simulink model "Exercicio_2_simulink_Vinicius"  (R2015a)
settings: Solver=ode45  StartTime=0.0  StopTime=40  RelTol=1e-3
values from neighbouring files (symbols this model uses):
  B = [zeros(1,d) 0.4 0.6]    [Exercicio_2_Vinicius_Alexandre.m]
  Ts = 1    [Exercicio_2_Vinicius_Alexandre.m]
undefined symbols (not defined in the file or in its folder): At, D, ke, kf, kw
settings Model: Creator=vinic  LastModifiedBy=vinic

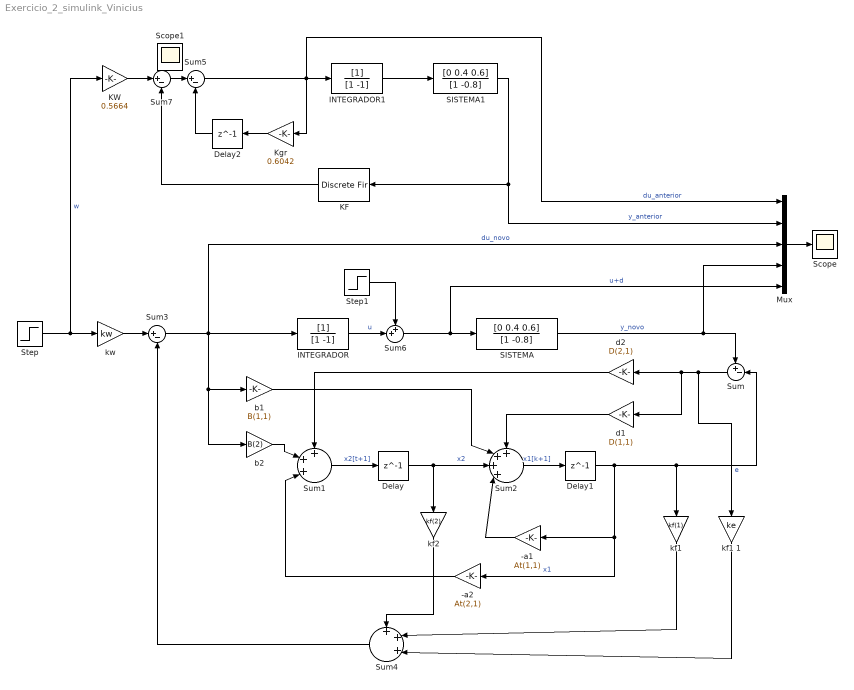
== system Exercicio_2_simulink_Vinicius ==
  -a1 : Gain  Gain=At(1,1)
  -a2 : Gain  Gain=At(2,1)
  Delay : Delay  DelayLength=1  SampleTime=Ts
  Delay1 : Delay  DelayLength=1  SampleTime=Ts
  Delay2 : Delay  DelayLength=1  SampleTime=Ts
  INTEGRADOR : DiscreteFilter  Denominator=[1 -1]  SampleTime=Ts
  INTEGRADOR1 : DiscreteFilter  Denominator=[1 -1]  SampleTime=Ts
  KF : DiscreteFir  Coefficients=[1.372 -0.8056]  SampleTime=Ts
  KW : Gain  Gain=0.5664
  "Kgr " : Gain  Gain=0.6042
  Mux : Mux  Inputs=5
  SISTEMA : DiscreteFilter  Numerator=[0 0.4 0.6]  Denominator=[1 -0.8]  SampleTime=Ts
  SISTEMA1 : DiscreteFilter  Numerator=[0 0.4 0.6]  Denominator=[1 -0.8]  SampleTime=Ts
  Scope : Scope
      settings: ShowLegends=on  YMin=-0.2  YMax=1.2  SaveName=sld
  Step : Step  Time=0  SampleTime=Ts
  Step1 : Step  Time=15  After=0.1  SampleTime=Ts
  Sum : Sum  Inputs=+-|
  Sum1 : Sum  Inputs=+++|
  Sum2 : Sum  Inputs=++++|
  Sum3 : Sum  Inputs=|+-
  Sum4 : Sum  Inputs=+++|
  Sum5 : Sum  Inputs=|+-
  Sum6 : Sum  Inputs=++|
  Sum7 : Sum  Inputs=|+-
  b1 : Gain  Gain=B(1,1)
  b2 : Gain  Gain=B(2)
  d1 : Gain  Gain=D(1,1)
  d2 : Gain  Gain=D(2,1)
  "kf1 " : Gain  Gain=kf(1)
  kf1 1 : Gain  Gain=ke
  kf2 : Gain  Gain=kf(2)
  "kw " : Gain  Gain=kw
  Scope1 : Scope
  wires:
  SISTEMA/1 -> Mux/4, Sum/1  "y_novo"
  Sum3/1 -> Mux/3, INTEGRADOR/1, b2/1, b1/1  "du_novo"
  Sum1/1 -> Delay/1  "x2[t+1]"
  Delay/1 -> kf2/1, Sum2/3  "x2"
  Sum2/1 -> Delay1/1  "x1[k+1]"
  b2/1 -> Sum1/2
  b1/1 -> Sum2/2
  Delay1/1 -> -a2/1, -a1/1, Sum/2, "kf1 "/1  "x1"
  -a1/1 -> Sum2/4
  -a2/1 -> Sum1/3
  Sum/1 -> kf1 1/1, d1/1, d2/1  "e"
  d2/1 -> Sum1/1
  d1/1 -> Sum2/1
  "kw "/1 -> Sum3/1
  kf2/1 -> Sum4/1
  "kf1 "/1 -> Sum4/2
  kf1 1/1 -> Sum4/3
  Sum4/1 -> Sum3/2
  Mux/1 -> Scope/1
  SISTEMA1/1 -> Mux/2, KF/1  "y_anterior"
  Step/1 -> KW/1, "kw "/1  "w"
  KF/1 -> Sum7/2
  KW/1 -> Sum7/1
  INTEGRADOR1/1 -> SISTEMA1/1
  "Kgr "/1 -> Delay2/1
  Delay2/1 -> Sum5/2
  Sum7/1 -> Sum5/1
  Sum5/1 -> Mux/1, "Kgr "/1, INTEGRADOR1/1  "du_anterior"
  INTEGRADOR/1 -> Sum6/2  "u"
  Sum6/1 -> Mux/5, SISTEMA/1  "u+d"
  Step1/1 -> Sum6/1
